simulink model "test_stateflow"  (R2015b)
settings: Solver=FixedStepAuto  StartTime=0.0  StopTime=10.0  FixedStep=0.001  RelTol=1e-3
settings Model: Creator=rcasado  LastModifiedBy=rcasado

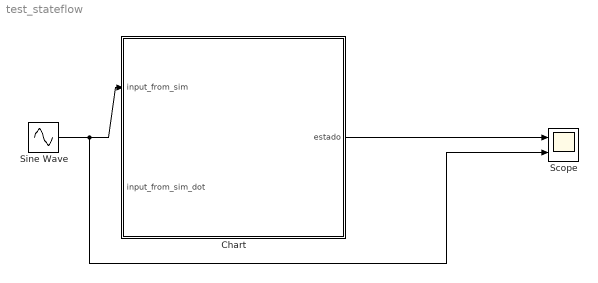
== system test_stateflow ==
  Chart : Stateflow chart  TreatAsAtomicUnit=on
  Scope : Scope  NumInputPorts=2
  Sine Wave : Sin  Amplitude=5  SampleTime=0
  wires:
  Chart/1(estado) -> Scope/1
  Sine Wave/1 -> Scope/2, Chart/1(input_from_sim)

== stateflow chart test_stateflow/Chart ==
  settings: updateMethod=CONTINUOUS
  state subiendo
    entry:
    estado = 1;
    during:
  state bajando
    entry:
    estado = -1;
    during:
  (default) -> subiendo
  subiendo -> bajando : [input < 0]
  bajando -> subiendo : [input_from_sim > 0]
  data: input_from_sim input; estado output; input_from_sim_dot input; input local
  data input settings: updateMethod=SF_CONTINUOUS_TIME_DATA
